simulink model "scott_connection"  (R2020a)
settings: Solver=VariableStepAuto  StartTime=0.0  StopTime=10.0  RelTol=1e-3
libraries: powerlib x12, powerlib_meascontrol x5
settings Model: Creator=Manisha  LastModifiedBy=Manisha

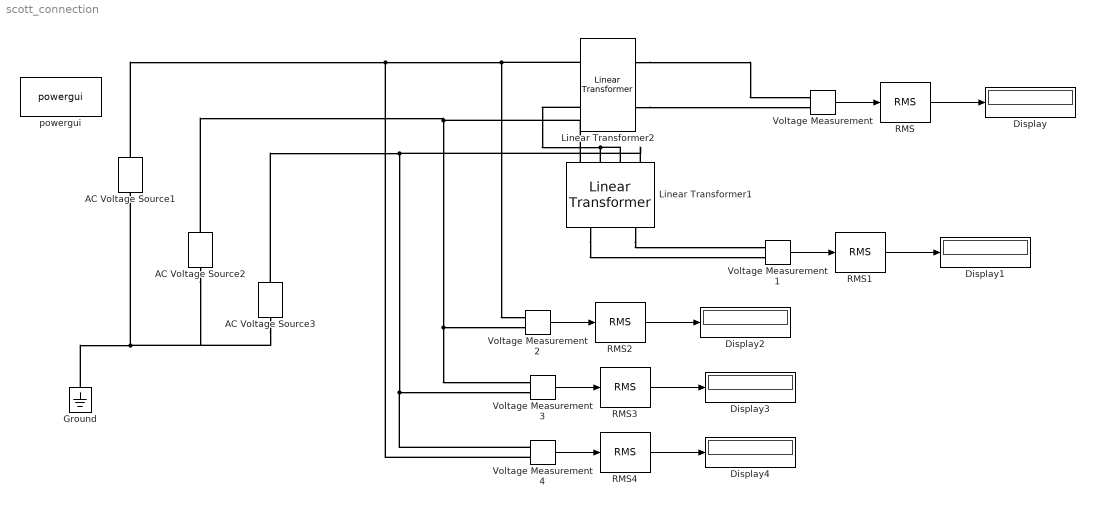
== system scott_connection ==
  AC Voltage Source1 : powerlib/Electrical Sources/AC Voltage Source  Amplitude=230*1.414  Phase=0  Frequency=50  SampleTime=0  Measurements=Voltage  BusType=swing  Pref=10e3  Qref=0  Qmin=-inf  Qmax=+inf
  AC Voltage Source2 : powerlib/Electrical Sources/AC Voltage Source  Amplitude=230*1.414  Phase=120  Frequency=50  SampleTime=0  Measurements=Voltage  BusType=swing  Pref=10e3  Qref=0  Qmin=-inf  Qmax=+inf
  AC Voltage Source3 : powerlib/Electrical Sources/AC Voltage Source  Amplitude=230*1.414  Phase=240  Frequency=50  SampleTime=0  Measurements=Voltage  BusType=swing  Pref=10e3  Qref=0  Qmin=-inf  Qmax=+inf
  Display{,1..4} (5 alike) : Display
  Ground : powerlib/Elements/Ground  LConnTagsString=a
  Linear Transformer1 : powerlib/Elements/Linear Transformer  UNITS=SI  NominalPower=[25000 50 ]  winding1=[800 0.007488 0.0000319]  winding2=[200 0.7488 0.00319]  ThreeWindings=on  winding3=[200 0.7488 0.00319]  RmLm=[33391 15.9409]  Measurements=None  DataType=on
  Linear Transformer2 : powerlib/Elements/Linear Transformer  UNITS=SI  NominalPower=[25000 50 ]  winding1=[400*0.866 0.7488 0.00319]  winding2=[800 0.007488 0.0000319]  ThreeWindings=off  winding3=[3.15e+05 3969 505.35]  RmLm=[33391 15.9409]  Measurements=None  DataType=on
  RMS{,1..4} (5 alike) : powerlib_meascontrol/Measurements/RMS  TrueRMS=on  Freq=50  RMSInit=120  Ts=0
  Voltage Measurement{,1..4} (5 alike) : powerlib/Measurements/Voltage Measurement  PhasorSimulation=off  OutputType=Complex  PSBequivalent=0
  powergui : powerlib/powergui  Priority=1  SimulationMode=Continuous  SampleTime=50e-6  frequency=60  Iterations=50  frequencyindice=50  Pbase=100e6  ErrMax=1e-4  UnitsV=kV  UnitsW=MW  buscounter=0  FunctionMessages=off  echomessages=off  EnableUseOfTLC=off  CurrentSourceSwitches=off  DisableSnubberDevices=off  DisableRonSwitches=off  DisableVfSwitches=off  DisplayEquations=off  AutomaticDiscreteSolvers=off  SolverType=Tustin/Backward Euler (TBE)  Interpol=off  ExternalGateDelay=off  methode=off  Ts=100  x0status=blocks  SPID=on  SwTol=0  HookPort=off  NonlinearTolerance=1e-4  nMaxIteration=100  ContinueOnMaxIteration=off  RestoreLinks=warning  ResistiveCurrentMeasurement=off  Frange=[0:2:500]  Ylog=off  Xlog=on  ShowGrid=off  save=off  variable=ZData  structure=0  ZoomFFT=off  StartTime=0.0  cycles=1  DisplayStyle=1  fundamental=60  FreqAxis=off  MaxFrequency=1000  frequencyindicesteady=1  RmsSteady=1  display=off
  wires:
  RMS/1 -> Display/1
  Voltage Measurement/1 -> RMS/1
  RMS1/1 -> Display1/1
  Voltage Measurement1/1 -> RMS1/1
  RMS2/1 -> Display2/1
  Voltage Measurement2/1 -> RMS2/1
  RMS3/1 -> Display3/1
  Voltage Measurement3/1 -> RMS3/1
  RMS4/1 -> Display4/1
  Voltage Measurement4/1 -> RMS4/1
  connections:
  Ground/LConn1 -- AC Voltage Source3/LConn1 -- AC Voltage Source2/LConn1 -- AC Voltage Source1/LConn1
  Linear Transformer2/RConn1 -- Voltage Measurement/LConn1
  Linear Transformer2/RConn2 -- Voltage Measurement/LConn2
  Linear Transformer1/RConn3 -- Linear Transformer2/LConn2 -- Linear Transformer1/RConn2
  AC Voltage Source1/RConn1 -- Voltage Measurement4/LConn2 -- Linear Transformer2/LConn1 -- Voltage Measurement2/LConn1
  AC Voltage Source3/RConn1 -- Linear Transformer1/RConn4 -- Voltage Measurement4/LConn1 -- Voltage Measurement3/LConn2
  AC Voltage Source2/RConn1 -- Voltage Measurement2/LConn2 -- Voltage Measurement3/LConn1 -- Linear Transformer1/RConn1
  Linear Transformer1/LConn2 -- Voltage Measurement1/LConn1
  Linear Transformer1/LConn1 -- Voltage Measurement1/LConn2
